simulink model "UAM_FlightModeManager"  (R2024b)
settings: Solver=FixedStepAuto  StartTime=0.0  StopTime=10.0  RelTol=1e-3
libraries: simulink x1
settings Model: DataDictionary=UAM_data.sldd  Creator=admin  LastModifiedBy=admin
settings OptimizationCC: DefaultParameterBehavior=Inlined  EnhancedBackFolding=on  PassReuseOutputArgsAs=Individual arguments  ZeroExternalMemoryAtStartup=off  ZeroInternalMemoryAtStartup=off  OptimizeBlockOrder=speed  DifferentSizesBufferReuse=on  OptimizationCustomize=off  EfficientTunableParamExpr=on
settings DebuggingCC: ParameterTunabilityLossMsg=error
settings HardwareCC: ProdBitPerLong=64  ProdLargestAtomicInteger=LongLong  ProdLargestAtomicFloat=Double  ProdLongLongMode=on  ProdHWDeviceType=ARM Compatible->ARM Cortex-A (64-bit)
settings SFSimCC: MATLABDynamicMemAlloc=off
settings RTWCC: Description=Embedded Coder  SystemTargetFile=ert.tlc  TemplateMakefile=ert_default_tmf  Toolchain=Linaro AArch64 Linux v6.3.1
settings CodeAppCC: ForceParamTrailComments=on  IgnoreCustomStorageClasses=off  OperatorAnnotations=on  SimulinkDataObjDesc=on  SFDataObjDesc=on  CustomSymbolStrGlobalVar=MGR_$N$M  CustomSymbolStrType=MGR_$N$M_T  CustomSymbolStrField=MGR_$N$M  CustomSymbolStrFcn=MGR_$N$M$F  CustomSymbolStrBlkIO=MGR_rtb_$N$M  CustomSymbolStrTmpVar=MGR_tmp_$N$M  CustomSymbolStrMacro=MGR_$N$M_MACRO  InsertBlockDesc=on
settings ERTTargetCC: TargetLangStandard=C99 (ISO)  GenerateSampleERTMain=on  ERTCustomFileTemplate=example_file_process.tlc

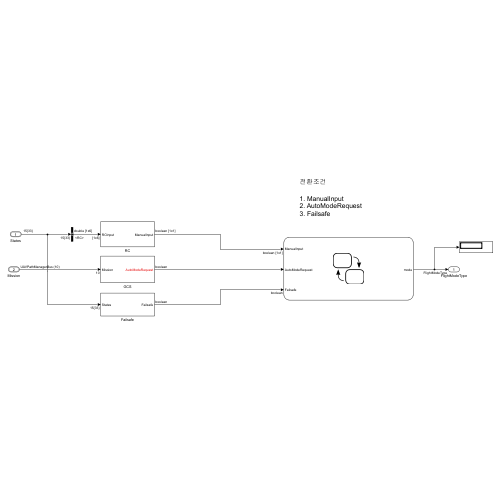
[thumbnail: Simulink's stored preview of the top-level diagram]
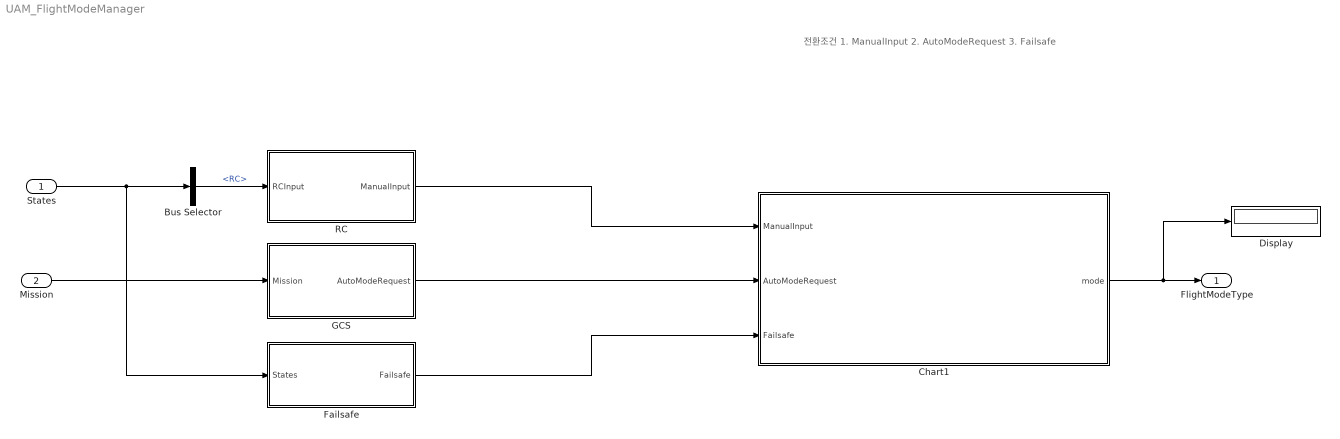
== system UAM_FlightModeManager ==
  note: 전환조건
      |
      | 1. ManualInput
      | 2. AutoModeRequest
      | 3. Failsafe
  States : Inport  OutDataTypeStr=Bus: sensorData
  Mission : Inport  Port=2  OutDataTypeStr=Bus: UAVPathManagerBus  PortDimensions=10  BusOutputAsStruct=on
  Bus Selector : BusSelector  OutputSignals=RC
  Chart1 : Stateflow chart  TreatAsAtomicUnit=on
      settings: PortSchema="{\"entries\":[{\"content\":{\"sides\":[{\"content\":{\"connectorIds\":[\"In2\",\"In3\",\"In1\"]},\"type\":\"ConnectorPlacement.EquallySpacedRectSide\",\"uuid\":\"7f808d98-1a22-47cf-b619-3081c4328c1f\"},{\"content\":{\"connectorIds\":[\"Out1\"],\"side\":\"RIGHT\"},\"type\":\"ConnectorPlacement.EquallySpacedRectSide\",\"uuid\":\"ee1ebc53-214f-4f44-afa8-7e67f94c306f\"},{\"content\":{\"side\":\"TOP\"},\"type\":\"ConnectorPlacement.EquallySpacedRectSide\",\"uuid\":\"a218192b-9bc0-4f77-b8de-414c3f6a9dd6\"}]},\"type\":\"ConnectorPlacement.EquallySpacedConnector\",\"uuid\":\"d7f6b7da-8a65-4043-9f4e-f6645b75040a\"}],\"packageUris\":[\"http://schema.mathworks.com/mf0/Connector/R2020b\"],\"version\":\"1.0\"}"
  Display : Display
  Failsafe : Subsystem
  GCS : Subsystem
  RC : Subsystem
  FlightModeType : Outport  OutDataTypeStr=Enum: FlightModeType
  wires:
  RC/1(ManualInput) -> Chart1/2(ManualInput)
  States/1 -> Failsafe/1(States), Bus Selector/1
  Chart1/1(mode) -> Display/1, FlightModeType/1
  Failsafe/1(Failsafe) -> Chart1/1(Failsafe)
  Bus Selector/1 -> RC/1(RCInput)  "<RC>"
  GCS/1(AutoModeRequest) -> Chart1/3(AutoModeRequest)
  Mission/1 -> GCS/1(Mission)

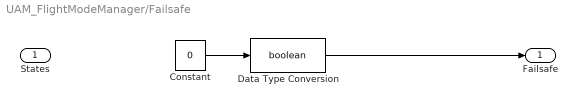
== system UAM_FlightModeManager/Failsafe ==
  States : Inport
  Constant : Constant  Value=0
  Data Type Conversion : DataTypeConversion  OutDataTypeStr=boolean  SaturateOnIntegerOverflow=off  RndMeth=Floor
  Failsafe : Outport  OutDataTypeStr=boolean  PortDimensions=1
  wires:
  Constant/1 -> Data Type Conversion/1
  Data Type Conversion/1 -> Failsafe/1

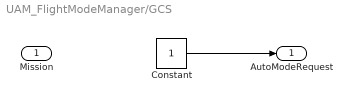
== system UAM_FlightModeManager/GCS ==
  Mission : Inport  OutDataTypeStr=Bus: UAVPathManagerBus
  Constant : Constant  OutDataTypeStr=boolean
  AutoModeRequest : Outport  OutDataTypeStr=boolean
  wires:
  Constant/1 -> AutoModeRequest/1

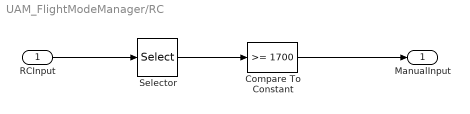
== system UAM_FlightModeManager/RC ==
  RCInput : Inport
  Compare To Constant : simulink/Logic and Bit Operations/Compare To Constant  relop=>=  const=1700  OutDataTypeStr=boolean
  Selector : Selector  InputPortWidth=6  IndexOptions=Index vector (dialog)  Indices=6  OutputSizes=1
  ManualInput : Outport  OutDataTypeStr=boolean
  wires:
  RCInput/1 -> Selector/1
  Compare To Constant/1 -> ManualInput/1
  Selector/1 -> Compare To Constant/1

== stateflow chart UAM_FlightModeManager/Chart1 ==
  state ManualState
    mode = FlightModeType.Manual;
  state AutoState
    mode = FlightModeType.Auto;
  state EmergecnyState
    mode = FlightModeType.Emergecny;
  (default) -> ManualState
  ManualState -> AutoState [order 1] : [AutoModeRequest && ~Failsafe && ~ManualInput]
  AutoState -> ManualState [order 1] : [ManualInput && ~Failsafe]
  ManualState -> EmergecnyState [order 2] : [Failsafe]
  EmergecnyState -> ManualState [order 1] : [[ManualInput && ~Failsafe]]
  AutoState -> EmergecnyState [order 2] : [Failsafe]
  EmergecnyState -> AutoState [order 2] : [[AutoModeRequest && ~Failsafe]]
  data: mode output Enum: FlightModeType; Failsafe input; ManualInput input; AutoModeRequest input
